simulink model "massSpring"  (R2024a)
settings: Solver=VariableStepAuto  StartTime=0.0  StopTime=500  RelTol=1e-3
model workspace (MAT data in the model file):
  C = 1
undefined symbols (not defined in the file): displacement, k, mass
settings Model: Creator=omar_  LastModifiedBy=omar_

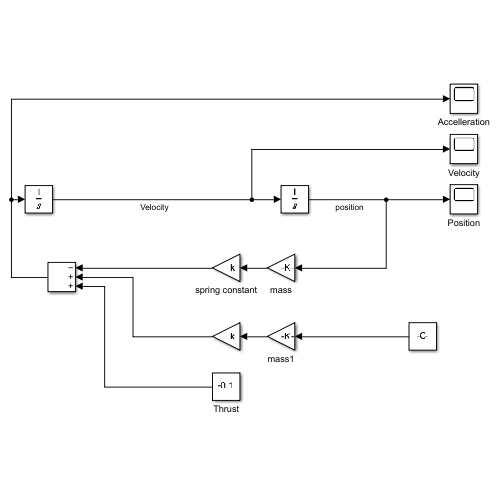
[thumbnail: Simulink's stored preview of the top-level diagram]
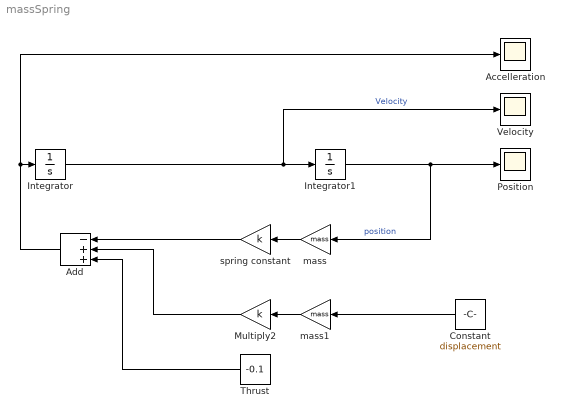
== system massSpring ==
  Accelleration : Scope
  Add : Sum  Inputs=-++
  Constant : Constant  Value=displacement
  Integrator : Integrator
  Integrator1 : Integrator
  Multiply2 : Gain  Gain=k
  Position : Scope
  Thrust : Constant  Value=-0.1
  Velocity : Scope
  mass : Gain  Gain=mass
  mass1 : Gain  Gain=mass
  spring constant : Gain  Gain=k
  wires:
  Integrator/1 -> Velocity/1, Integrator1/1  "Velocity"
  Integrator1/1 -> mass/1, Position/1  "position"
  mass/1 -> spring constant/1
  spring constant/1 -> Add/1
  Add/1 -> Accelleration/1, Integrator/1
  mass1/1 -> Multiply2/1
  Multiply2/1 -> Add/2
  Constant/1 -> mass1/1
  Thrust/1 -> Add/3
